simulink model "sampleModel2078"  (R2023a)
settings: Solver=VariableStepAuto  StartTime=0.0  StopTime=10.0  RelTol=1e-3
libraries: hdlsllib x5, simulink x2
settings Model: Creator=user1  LastModifiedBy=user1

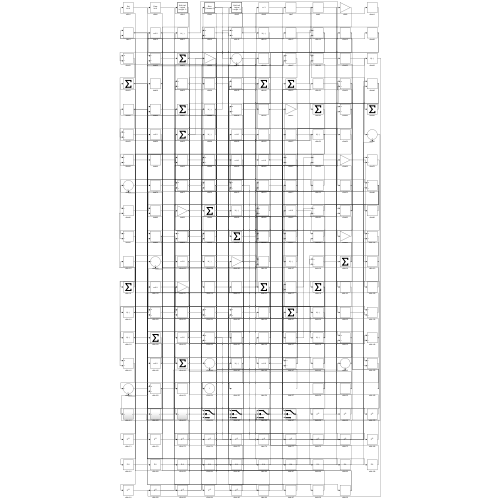
[thumbnail: Simulink's stored preview of the top-level diagram]
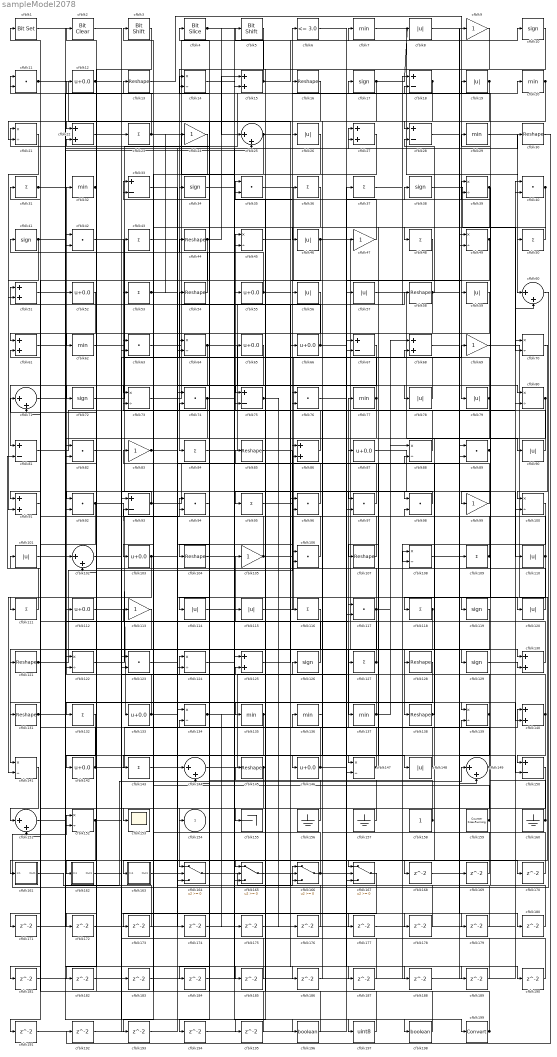
== system sampleModel2078 ==
  cfblk1 : simulink/Logic and Bit Operations/Bit Set  iBit=0
      settings: LibrarySourceBlock=|
      | hdlsllib/Logic and Bit
      | Operations/Bit Set
  cfblk{10,17,34,38,41,72,119,126,129} (9 alike) : Signum
  cfblk{14,21,39,45,49,64,70,73,80,88,100,108,122,124,134,139,141,147,152} (19 alike) : Product  Inputs=*/  RndMeth=Zero  SaturateOnIntegerOverflow=on
  cfblk{8,19,26,46,56..57,59,78..79,90,101,110,114..115,120,148} (16 alike) : Abs  SaturateOnIntegerOverflow=off
  cfblk{25,60,71,102,144,149,151} (7 alike) : Sum  Inputs=|++
  cfblk{12,52,55,65..66,87,103,112,133,142,146} (11 alike) : Bias  Bias=0.0  SaturateOnIntegerOverflow=off
  cfblk{13,16,30,44,54,58,85,104,107,121,128,131,138,145} (14 alike) : Reshape
  cfblk{9,24,47,69,83,99,105,113} (8 alike) : Gain
  cfblk{11,35,40,42,63,74,76,82,89,92,94,96..98,106,117,123} (17 alike) : DotProduct  OutDataTypeStr=Inherit: Inherit via internal rule
  cfblk{23,31,36..37,43,48,50,53,84,95,109,111,116,118,127,132,143} (17 alike) : Sum  Inputs=+
  cfblk{15,22,27,51,61,68,86,91,125,130,140} (11 alike) : Sum
  cfblk{7,20,29,32,62,77,135..137} (9 alike) : MinMax
  cfblk{18,28,33,67,75,81,93,150} (8 alike) : Sum  Inputs=+-
  cfblk153 : Scope
  cfblk155 : Terminator
  cfblk156 : Ground
  cfblk157 : Ground
  cfblk158 : Constant  SampleTime=-1
  cfblk159 : hdlsllib/Sources/Counter Free-Running  NumBits=16  tsamp=-1
  cfblk160 : Ground
  cfblk161 : Subsystem
      settings: LibrarySourceBlock=|
      | hdlsllib/Ports &
      | Subsystems/Subsystem
  cfblk162 : Subsystem
      settings: LibrarySourceBlock=|
      | hdlsllib/Ports &
      | Subsystems/Subsystem
  cfblk163 : Subsystem
      settings: LibrarySourceBlock=|
      | hdlsllib/Ports &
      | Subsystems/Subsystem
  cfblk{164..167} (4 alike) : Switch  SaturateOnIntegerOverflow=off  InputSameDT=off
  cfblk{168..195} (28 alike) : Delay  SampleTime=1
  cfblk196 : DataTypeConversion  OutDataTypeStr=boolean  SaturateOnIntegerOverflow=off  RndMeth=Floor
  cfblk197 : DataTypeConversion  OutDataTypeStr=uint8  SaturateOnIntegerOverflow=off  RndMeth=Floor
  cfblk198 : DataTypeConversion  OutDataTypeStr=boolean  SaturateOnIntegerOverflow=off  RndMeth=Floor
  cfblk199 : DataTypeConversion  SaturateOnIntegerOverflow=off  RndMeth=Floor
  cfblk2 : simulink/Logic and Bit Operations/Bit Clear  iBit=0
      settings: LibrarySourceBlock=|
      | hdlsllib/Logic and Bit
      | Operations/Bit Clear
  cfblk3 : hdlsllib/Logic and Bit Operations/Bit Shift  mode=Shift Left Logical  N=0
  cfblk4 : hdlsllib/Logic and Bit Operations/Bit Slice  lidx=7  ridx=0
  cfblk5 : hdlsllib/Logic and Bit Operations/Bit Shift  mode=Shift Left Logical  N=0
  cfblk6 : hdlsllib/Logic and Bit Operations/Compare To Constant  relop=<=  const=3.0  OutDataTypeStr=boolean
  cfblk154 : Outport  VectorParamsAs1DForOutWhenUnconnected=off
  wires:
  cfblk5/1 -> cfblk84/1
  cfblk13/1 -> cfblk79/1
  cfblk56/1 -> cfblk104/1
  cfblk54/1 -> cfblk32/1
  cfblk115/1 -> cfblk69/1
  cfblk93/1 -> cfblk49/1, cfblk92/1
  cfblk137/1 -> cfblk42/1, cfblk68/1
  cfblk63/1 -> cfblk10/1
  cfblk46/1 -> cfblk130/1, cfblk63/2
  cfblk148/1 -> cfblk77/1, cfblk41/1
  cfblk44/1 -> cfblk15/1, cfblk191/1
  cfblk130/1 -> cfblk102/1
  cfblk27/1 -> cfblk34/1
  cfblk76/1 -> cfblk38/1
  cfblk69/1 -> cfblk163/1(In1)
  cfblk139/1 -> cfblk126/1, cfblk165/2
  cfblk74/1 -> cfblk162/1(In1), cfblk36/1
  cfblk65/1 -> cfblk81/1
  cfblk98/1 -> cfblk95/1
  cfblk141/1 -> cfblk151/1
  cfblk161/1(Out1) -> cfblk149/1
  cfblk92/1 -> cfblk133/1, cfblk111/1
  cfblk64/1 -> cfblk80/1, cfblk131/1
  cfblk57/1 -> cfblk90/1
  cfblk122/1 -> cfblk94/1
  cfblk121/1 -> cfblk6/1, cfblk140/2
  cfblk158/1 -> cfblk21/1, cfblk73/2
  cfblk70/1 -> cfblk100/1
  cfblk37/1 -> cfblk19/1
  cfblk119/1 -> cfblk141/1
  cfblk49/1 -> cfblk147/1, cfblk167/2
  cfblk60/1 -> cfblk152/1
  cfblk145/1 -> cfblk155/1, cfblk35/2
  cfblk149/1 -> cfblk164/1, cfblk127/1, cfblk53/1
  cfblk90/1 -> cfblk45/1
  cfblk23/1 -> cfblk11/1, cfblk65/1
  cfblk134/1 -> cfblk26/1, cfblk175/1
  cfblk77/1 -> cfblk4/1, cfblk117/2
  cfblk3/1 -> cfblk72/1
  cfblk40/1 -> cfblk97/1, cfblk73/1
  cfblk7/1 -> cfblk60/1
  cfblk162/1(Out1) -> cfblk125/2
  cfblk58/1 -> cfblk121/1, cfblk61/1, cfblk28/2, cfblk150/2
  cfblk29/1 -> cfblk50/1
  cfblk132/1 -> cfblk142/1
  cfblk22/1 -> cfblk23/1
  cfblk9/1 -> cfblk15/2
  cfblk84/1 -> cfblk56/1
  cfblk96/1 -> cfblk14/1
  cfblk59/1 -> cfblk91/1
  cfblk144/1 -> cfblk37/1
  cfblk14/1 -> cfblk139/1
  cfblk86/1 -> cfblk76/1
  cfblk100/1 -> cfblk108/2
  cfblk131/1 -> cfblk51/1, cfblk165/3
  cfblk15/1 -> cfblk5/1, cfblk7/1
  cfblk26/1 -> cfblk75/1
  cfblk126/1 -> cfblk105/1
  cfblk62/1 -> cfblk98/1
  cfblk78/1 -> cfblk54/1
  cfblk17/1 -> cfblk8/1, cfblk67/2
  cfblk41/1 -> cfblk51/2, cfblk124/2, cfblk186/1
  cfblk81/1 -> cfblk60/2
  cfblk105/1 -> cfblk9/1, cfblk128/1, cfblk92/2
  cfblk160/1 -> cfblk16/1, cfblk124/1
  cfblk109/1 -> cfblk13/1, cfblk61/2
  cfblk110/1 -> cfblk118/1, cfblk94/2
  cfblk72/1 -> cfblk17/1
  cfblk147/1 -> cfblk87/1, cfblk33/2
  cfblk18/1 -> cfblk46/1, cfblk194/1
  cfblk85/1 -> cfblk116/1
  cfblk151/1 -> cfblk117/1
  cfblk89/1 -> cfblk29/1, cfblk39/2
  cfblk164/1 -> cfblk166/1
  cfblk138/1 -> cfblk98/2, cfblk88/2
  cfblk16/1 -> cfblk22/1
  cfblk117/1 -> cfblk71/1, cfblk88/1, cfblk172/1
  cfblk53/1 -> cfblk78/1, cfblk24/1
  cfblk48/1 -> cfblk107/1
  cfblk118/1 -> cfblk137/1, cfblk167/3
  cfblk45/1 -> cfblk66/1
  cfblk42/1 -> cfblk149/2
  cfblk146/1 -> cfblk39/1, cfblk136/1
  cfblk32/1 -> cfblk102/2, cfblk12/1
  cfblk73/1 -> cfblk18/1
  cfblk38/1 -> cfblk70/2
  cfblk39/1 -> cfblk99/1, cfblk165/1
  cfblk111/1 -> cfblk81/2
  cfblk125/1 -> cfblk58/1
  cfblk133/1 -> cfblk112/1, cfblk27/2
  cfblk52/1 -> cfblk152/2
  cfblk91/1 -> cfblk151/2
  cfblk113/1 -> cfblk161/1(In1)
  cfblk21/1 -> cfblk91/2
  cfblk33/1 -> cfblk106/1
  cfblk71/1 -> cfblk27/1
  cfblk80/1 -> cfblk119/1, cfblk123/2, cfblk82/2
  cfblk142/1 -> cfblk40/1, cfblk101/1
  cfblk47/1 -> cfblk35/1
  cfblk79/1 -> cfblk3/1, cfblk168/1
  cfblk107/1 -> cfblk86/1
  cfblk166/1 -> cfblk47/1, cfblk63/1
  cfblk19/1 -> cfblk146/1, cfblk28/1
  cfblk127/1 -> cfblk52/1, cfblk71/2
  cfblk163/1(Out1) -> cfblk85/1
  cfblk55/1 -> cfblk11/2, cfblk177/1
  cfblk103/1 -> cfblk134/1, cfblk141/2
  cfblk112/1 -> cfblk138/1
  cfblk123/1 -> cfblk144/1
  cfblk4/1 -> cfblk129/1, cfblk25/1
  cfblk94/1 -> cfblk64/1
  cfblk99/1 -> cfblk83/1
  cfblk87/1 -> cfblk110/1
  cfblk67/1 -> cfblk132/1
  cfblk129/1 -> cfblk130/2
  cfblk36/1 -> cfblk135/1
  cfblk136/1 -> cfblk106/2
  cfblk25/1 -> cfblk59/1, cfblk184/1
  cfblk50/1 -> cfblk48/1
  cfblk95/1 -> cfblk57/1
  cfblk1/1 -> cfblk199/1
  cfblk114/1 -> cfblk30/1
  cfblk152/1 -> cfblk82/1, cfblk68/2, cfblk181/1
  cfblk28/1 -> cfblk20/1
  cfblk75/1 -> cfblk55/1, cfblk176/1
  cfblk156/1 -> cfblk145/1
  cfblk35/1 -> cfblk89/1
  cfblk106/1 -> cfblk44/1
  cfblk31/1 -> cfblk148/1, cfblk188/1
  cfblk12/1 -> cfblk62/1, cfblk97/2
  cfblk11/1 -> cfblk96/1, cfblk25/2
  cfblk143/1 -> cfblk140/1
  cfblk20/1 -> cfblk21/2, cfblk114/1
  cfblk66/1 -> cfblk31/1, cfblk189/1
  cfblk88/1 -> cfblk43/1
  cfblk24/1 -> cfblk143/1
  cfblk120/1 -> cfblk22/2
  cfblk97/1 -> cfblk74/2
  cfblk101/1 -> cfblk18/2
  cfblk135/1 -> cfblk153/1, cfblk75/2
  cfblk108/1 -> cfblk109/1
  cfblk61/1 -> cfblk167/1
  cfblk157/1 -> cfblk33/1
  cfblk159/1 -> cfblk113/1, cfblk154/1
  cfblk83/1 -> cfblk103/1, cfblk120/1
  cfblk140/1 -> cfblk150/1, cfblk122/2
  cfblk168/1 -> cfblk49/2
  cfblk8/1 -> cfblk169/1
  cfblk169/1 -> cfblk76/2
  cfblk6/1 -> cfblk170/1
  cfblk170/1 -> cfblk67/1
  cfblk150/1 -> cfblk171/1
  cfblk171/1 -> cfblk42/2
  cfblk172/1 -> cfblk80/2
  cfblk116/1 -> cfblk173/1
  cfblk173/1 -> cfblk122/1
  cfblk43/1 -> cfblk174/1
  cfblk174/1 -> cfblk125/1
  cfblk175/1 -> cfblk70/1
  cfblk176/1 -> cfblk134/2
  cfblk177/1 -> cfblk40/2
  cfblk104/1 -> cfblk178/1
  cfblk178/1 -> cfblk74/1
  cfblk82/1 -> cfblk179/1
  cfblk179/1 -> cfblk166/2
  cfblk68/1 -> cfblk180/1
  cfblk180/1 -> cfblk139/2
  cfblk128/1 -> cfblk182/1
  cfblk182/1 -> cfblk100/2
  cfblk102/1 -> cfblk183/1
  cfblk183/1 -> cfblk108/1
  cfblk184/1 -> cfblk45/2
  cfblk51/1 -> cfblk185/1
  cfblk185/1 -> cfblk123/1
  cfblk186/1 -> cfblk166/3
  cfblk124/1 -> cfblk187/1
  cfblk187/1 -> cfblk86/2
  cfblk188/1 -> cfblk89/2
  cfblk189/1 -> cfblk144/2
  cfblk165/1 -> cfblk190/1
  cfblk190/1 -> cfblk96/2
  cfblk191/1 -> cfblk64/2
  cfblk30/1 -> cfblk192/1
  cfblk192/1 -> cfblk93/1
  cfblk167/1 -> cfblk193/1
  cfblk193/1 -> cfblk164/3
  cfblk194/1 -> cfblk147/2
  cfblk10/1 -> cfblk195/1
  cfblk195/1 -> cfblk164/2
  cfblk34/1 -> cfblk196/1
  cfblk196/1 -> cfblk2/1
  cfblk2/1 -> cfblk197/1
  cfblk197/1 -> cfblk115/1
  cfblk181/1 -> cfblk198/1
  cfblk198/1 -> cfblk1/1
  cfblk199/1 -> cfblk14/2, cfblk93/2

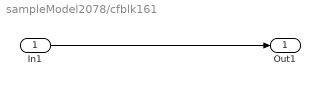
== system sampleModel2078/cfblk161 ==
  In1 : Inport
  Out1 : Outport
  wires:
  In1/1 -> Out1/1

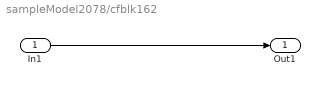
== system sampleModel2078/cfblk162 ==
  In1 : Inport
  Out1 : Outport
  wires:
  In1/1 -> Out1/1

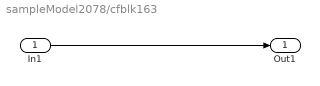
== system sampleModel2078/cfblk163 ==
  In1 : Inport
  Out1 : Outport
  wires:
  In1/1 -> Out1/1
